simulink model "hil"  (R2020a)
settings: Solver=FixedStepAuto  StartTime=0.0  StopTime=inf  RelTol=1e-3  EnableMultiTasking=on
values from neighbouring files (symbols this model uses):
  K_final = [0 0 0 0]    [lin_mod.m]    (also in lin_mod_param.mat; lqrr.m = K)
  refernce_values = [0; 0 ;0; 0]    [lin_mod.m]    (also in lin_mod_param.mat = [0 0 0 0]; lqrr.m = [0; 0;0;0 ])
libraries: arduinolib x3, eeGeneralControl x2
settings Model: SILPILModeSetting=veronly  ExtModeTrigDuration=2  Creator=mahmo  LastModifiedBy=mahmo
settings OptimizationCC: EnhancedBackFolding=on  PassReuseOutputArgsAs=Individual arguments  ZeroExternalMemoryAtStartup=off  ZeroInternalMemoryAtStartup=off  MaxStackSize=64  OptimizeBlockOrder=speed  DifferentSizesBufferReuse=on  OptimizationCustomize=off  EfficientTunableParamExpr=on
settings DebuggingCC: ParameterTunabilityLossMsg=error
settings HardwareCC: ProdBitPerInt=16  ProdBitPerPointer=16  ProdBitPerSizeT=16  ProdBitPerPtrDiffT=16  ProdLargestAtomicFloat=None  ProdWordSize=8  ProdHWDeviceType=Atmel->AVR
settings SFSimCC: MATLABDynamicMemAlloc=off
settings RTWCC: SystemTargetFile=ert.tlc  HardwareBoard=Arduino Mega 2560  TLCOptions=-aInlineSetEventsForThisBaseRateFcn=TLC_FALSE -aSuppressMultiTaskScheduler=TLC_FALSE -aRateBasedStepFcn=1  TemplateMakefile=ert_default_tmf  Toolchain=Arduino AVR  BuildConfiguration=Faster Runs
settings CodeAppCC: ForceParamTrailComments=on  IgnoreCustomStorageClasses=off  OperatorAnnotations=on  SimulinkDataObjDesc=on  SFDataObjDesc=on  InsertBlockDesc=on
settings ERTTargetCC: SupportContinuousTime=on  SupportVariableSizeSignals=on  ExtModeStaticAllocSize=2048

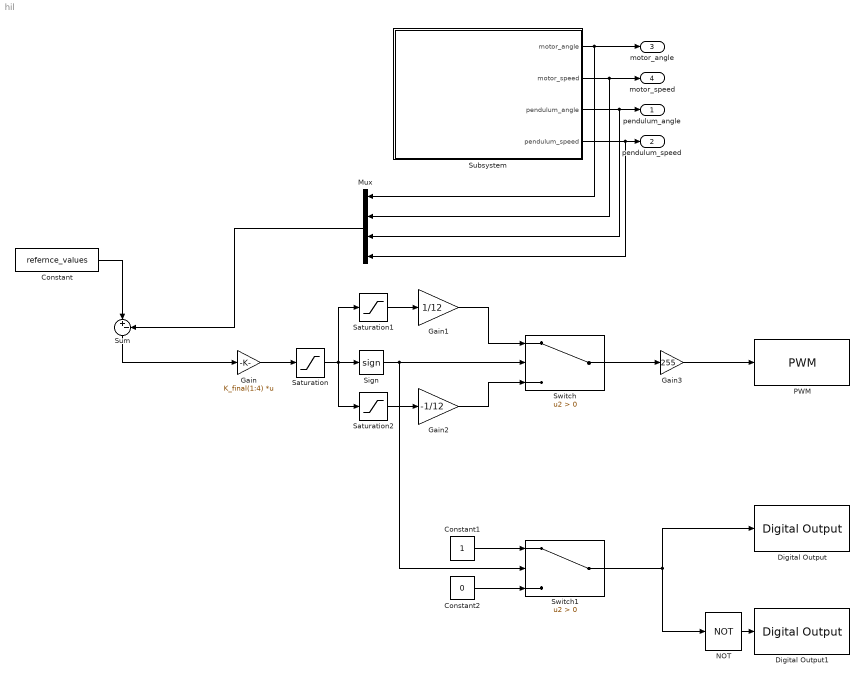
== system hil ==
  Constant : Constant  Value=refernce_values
  Constant1 : Constant
  Constant2 : Constant  Value=0
  Digital Output : arduinolib/Digital Output  pinNumber=7  Direction=output  blockPlatform=arduino
  Digital Output1 : arduinolib/Digital Output  pinNumber=8  Direction=output  blockPlatform=arduino
  Gain : Gain  Gain=K_final(1:4)  Multiplication=Matrix(K*u)
  Gain1 : Gain  Gain=1/12
  Gain2 : Gain  Gain=-1/12
  Gain3 : Gain  Gain=255
  Mux : Mux
  NOT : Logic  Operator=NOT  IconShape=distinctive  AllPortsSameDT=off  OutDataTypeStr=boolean
  PWM : arduinolib/PWM  pinNumber=5  frequencyType=Default  desiredFrequency=490.2  achievableFrequency=490.2
  Saturation : Saturate  UpperLimit=12  LowerLimit=-12
  Saturation1 : Saturate  UpperLimit=12  LowerLimit=5
  Saturation2 : Saturate  UpperLimit=-5  LowerLimit=-12
  Sign : Signum
  Subsystem : Subsystem
  Sum : Sum  Inputs=|+-
  Switch : Switch  Criteria=u2 > Threshold
  Switch1 : Switch  Criteria=u2 > Threshold
  pendulum_angle : Outport
  pendulum_speed : Outport  Port=2
  motor_angle : Outport  Port=3
  motor_speed : Outport  Port=4
  wires:
  Subsystem/1(motor_angle) -> Mux/1, motor_angle/1
  Subsystem/2(motor_speed) -> Mux/2, motor_speed/1
  Subsystem/3(pendulum_angle) -> Mux/3, pendulum_angle/1
  Subsystem/4(pendulum_speed) -> Mux/4, pendulum_speed/1
  Sum/1 -> Gain/1
  Constant/1 -> Sum/1
  Mux/1 -> Sum/2
  Gain/1 -> Saturation/1
  Saturation/1 -> Saturation1/1, Saturation2/1, Sign/1
  Sign/1 -> Switch1/2, Switch/2
  Gain1/1 -> Switch/1
  Gain2/1 -> Switch/3
  Switch/1 -> Gain3/1
  Switch1/1 -> Digital Output/1, NOT/1
  NOT/1 -> Digital Output1/1
  Constant1/1 -> Switch1/1
  Constant2/1 -> Switch1/3
  Gain3/1 -> PWM/1
  Saturation1/1 -> Gain1/1
  Saturation2/1 -> Gain2/1

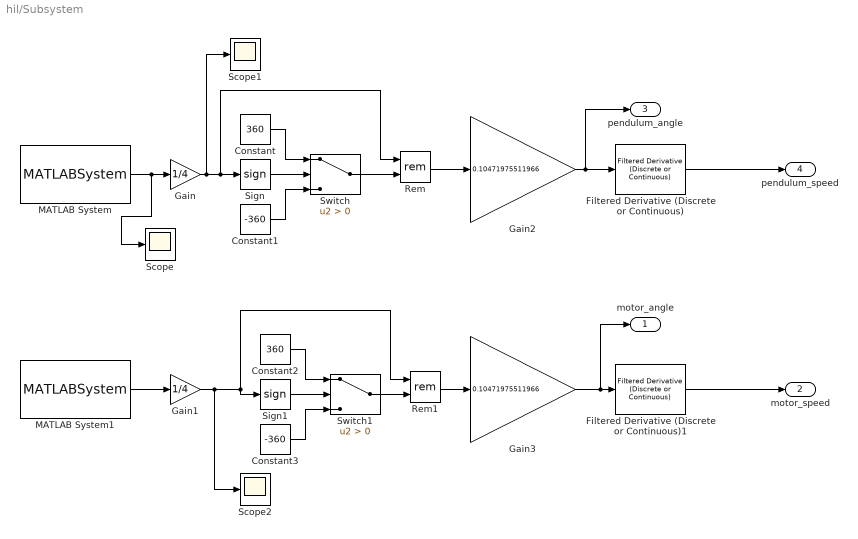
== system hil/Subsystem ==
  Constant : Constant  Value=360  OutDataTypeStr=double
  Constant1 : Constant  Value=-360  OutDataTypeStr=double
  Constant2 : Constant  Value=360  OutDataTypeStr=double
  Constant3 : Constant  Value=-360  OutDataTypeStr=double
  Filtered Derivative (Discrete or Continuous) : eeGeneralControl/Filtered Derivative (Discrete or Continuous)  K=1  T=0.1  B=inf  A=-inf  minRatio=10  init_option=Inherited from block input  x0=0  Ts=-1
      settings: SourceProductBaseCode=PS
  Filtered Derivative (Discrete or Continuous)1 : eeGeneralControl/Filtered Derivative (Discrete or Continuous)  K=1  T=0.1  B=inf  A=-inf  minRatio=10  init_option=Inherited from block input  x0=0  Ts=-1
      settings: SourceProductBaseCode=PS
  Gain : Gain  Gain=1/4  OutDataTypeStr=double
  Gain1 : Gain  Gain=1/4  OutDataTypeStr=double  RndMeth=Round
  Gain2 : Gain  Gain=0.10471975511966
  Gain3 : Gain  Gain=0.10471975511966
  MATLAB System : MATLABSystem  System=Encoder_arduino  Encoder=0  PinA=2  PinB=3  SampleTime=0.005
      mask Type: Encoder_arduino
      mask Display:
      | disp('Encoder');
      | port_label('output',1,'y');
  MATLAB System1 : MATLABSystem  System=Encoder_arduino  Encoder=0  PinA=20  PinB=21  SampleTime=0.005
      mask Type: Encoder_arduino
      mask Display:
      | disp('Encoder');
      | port_label('output',1,'y');
  Rem : Math  Operator=rem  SaturateOnIntegerOverflow=on
  Rem1 : Math  Operator=rem  SaturateOnIntegerOverflow=on
  Scope : Scope
  Scope1 : Scope
  Scope2 : Scope
  Sign : Signum
  Sign1 : Signum
  Switch : Switch  Criteria=u2 > Threshold
  Switch1 : Switch  Criteria=u2 > Threshold
  motor_angle : Outport
  motor_speed : Outport  Port=2
  pendulum_angle : Outport  Port=3
  pendulum_speed : Outport  Port=4
  wires:
  Gain1/1 -> Scope2/1, Sign1/1, Rem1/1
  Constant/1 -> Switch/1
  Rem1/1 -> Gain3/1
  Sign/1 -> Switch/2
  Rem/1 -> Gain2/1
  Constant3/1 -> Switch1/3
  Gain3/1 -> motor_angle/1, Filtered Derivative (Discrete or Continuous)1/1
  Gain2/1 -> pendulum_angle/1, Filtered Derivative (Discrete or Continuous)/1
  MATLAB System1/1 -> Gain1/1
  Constant1/1 -> Switch/3
  Filtered Derivative (Discrete or Continuous)/1 -> pendulum_speed/1
  Gain/1 -> Scope1/1, Rem/1, Sign/1
  MATLAB System/1 -> Scope/1, Gain/1
  Switch/1 -> Rem/2
  Filtered Derivative (Discrete or Continuous)1/1 -> motor_speed/1
  Sign1/1 -> Switch1/2
  Constant2/1 -> Switch1/1
  Switch1/1 -> Rem1/2
